simulink model "ex3"  (Simulink 6.0)
settings: Solver=ode45  StartTime=0.0  StopTime=10.0  RelTol=1e-3
settings Model: LastModifiedBy=lxy

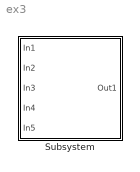
== system ex3 ==
  Subsystem : Subsystem

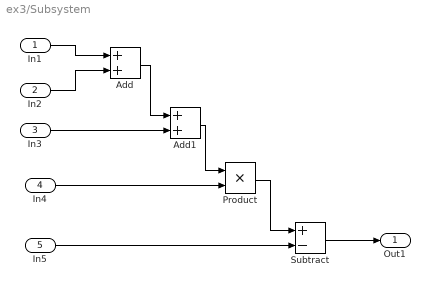
== system ex3/Subsystem ==
  In1 : Inport  Port=1  LatchInput=off
  In2 : Inport  Port=2  LatchInput=off
  In3 : Inport  Port=3  LatchInput=off
  In4 : Inport  Port=4  LatchInput=off
  In5 : Inport  Port=5  LatchInput=off
  Add : Sum  OutScaling=2^-10
  Add1 : Sum  OutScaling=2^-10
  Product : Product  RndMeth=Zero
  Subtract : Sum  Inputs=+-  OutScaling=2^-10
  Out1 : Outport
  wires:
  In1/1 -> Add/1
  In2/1 -> Add/2
  Add/1 -> Add1/1
  In3/1 -> Add1/2
  Add1/1 -> Product/1
  In4/1 -> Product/2
  Product/1 -> Subtract/1
  In5/1 -> Subtract/2
  Subtract/1 -> Out1/1
